simulink model "w3p1"  (R2020b)
settings: Solver=VariableStepAuto  StartTime=0.0  StopTime=10.0  RelTol=1e-3
settings Model: Creator=WELCOME  LastModifiedBy=WELCOME

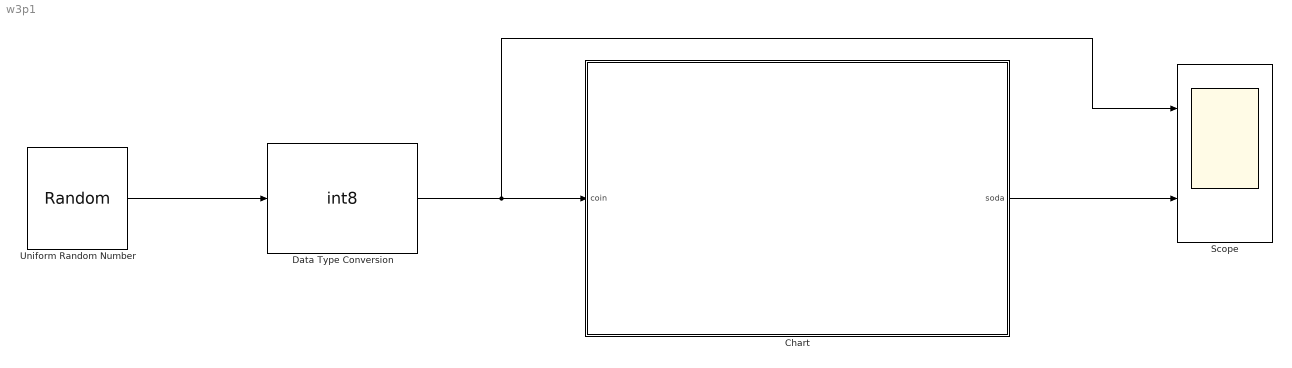
== system w3p1 ==
  Chart : Stateflow chart  TreatAsAtomicUnit=on
  Data Type Conversion : DataTypeConversion  OutDataTypeStr=int8  RndMeth=Nearest  SaturateOnIntegerOverflow=on
  Scope : Scope  NumInputPorts=2
  Uniform Random Number : UniformRandomNumber  SampleTime=0.1
  wires:
  Chart/1(soda) -> Scope/2
  Data Type Conversion/1 -> Scope/1, Chart/1(coin)
  Uniform Random Number/1 -> Data Type Conversion/1

== stateflow chart w3p1/Chart ==
  settings: stateMachineType=MEALY_MACHINE
  state got_0
  state got_nickel
  state got_dime
  (default) -> got_0
  got_0 -> got_nickel [order 1] : [coin==1]{soda=0}
  got_nickel -> got_0 [order 2] : [coin==2]{soda=1}
  got_nickel -> got_dime [order 1] : [coin==1]{soda=0}
  got_dime -> got_nickel [order 2] : [coin==2]{soda=1}
  got_dime -> got_0 [order 1] : [coin==1]{soda=1}
  got_0 -> got_dime [order 2] : [coin==2]{soda=0}
  data: coin input int8; soda output boolean
